simulink model "mdl_filter_kalmanIntegration_16b"  (R2016b)
settings: Solver=ode4  StartTime=0.0  StopTime=10.0  FixedStep=filterKalman_par.T  RelTol=1e-3
undefined symbols (not defined in the file or in its folder): Ag_phi_rad, Ag_theta_rad, AgVel_p_radPerScnd, AgVel_q_radPerScnd, filterKalman_par
settings Model: Creator=Nu  LastModifiedBy=Nu

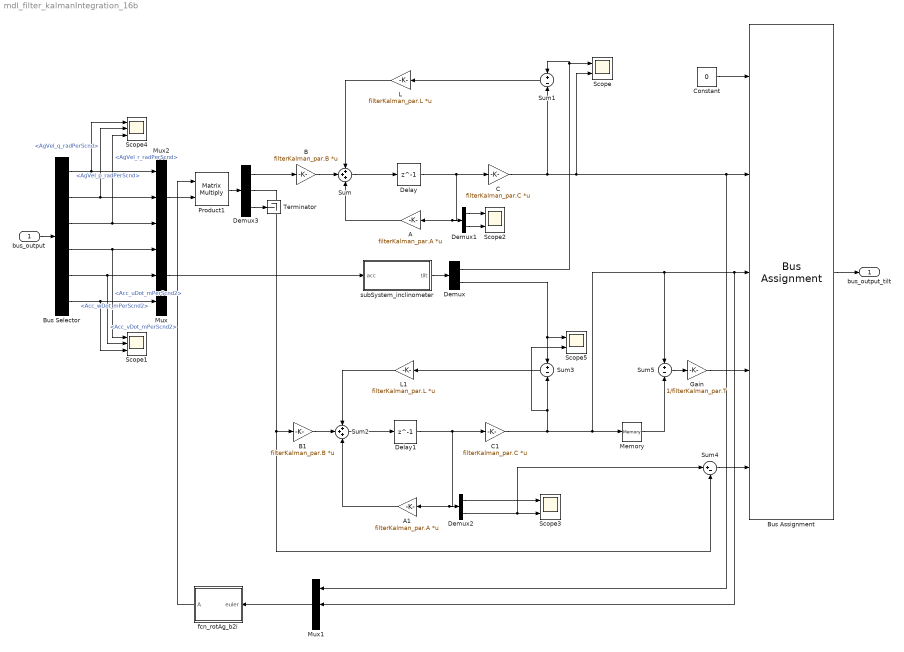
== system mdl_filter_kalmanIntegration_16b ==
  bus_output : Inport  OutDataTypeStr=Bus: mdl_output
  A : Gain  Gain=filterKalman_par.A  Multiplication=Matrix(K*u)
  A1 : Gain  Gain=filterKalman_par.A  Multiplication=Matrix(K*u)
  B : Gain  Gain=filterKalman_par.B  Multiplication=Matrix(K*u)
  B1 : Gain  Gain=filterKalman_par.B  Multiplication=Matrix(K*u)
  Bus Assignment : BusAssignment  AssignedSignals=Ag_phi_rad,Ag_theta_rad,AgVel_p_radPerScnd,AgVel_q_radPerScnd
  Bus Selector : BusSelector  OutputSignals=AgVel_p_radPerScnd,AgVel_q_radPerScnd,AgVel_r_radPerScnd,Acc_uDot_mPerScnd2,Acc_vDot_mPerScnd2,Acc_wDot_mPerScnd2
  C : Gain  Gain=filterKalman_par.C  Multiplication=Matrix(K*u)
  C1 : Gain  Gain=filterKalman_par.C  Multiplication=Matrix(K*u)
  Constant : Constant  Value=0  OutDataTypeStr=Bus: mdl_statesExt
  Delay : Delay  DelayLength=1  InitialCondition=[0 -0.014]
  Delay1 : Delay  DelayLength=1  InitialCondition=[0 -0.014]
  Demux : Demux  Outputs=2
  Demux1 : Demux  Outputs=2
  Demux2 : Demux  Outputs=2
  Demux3 : Demux  Outputs=3
  Gain : Gain  Gain=1/filterKalman_par.T
  L : Gain  Gain=filterKalman_par.L  Multiplication=Matrix(K*u)
  L1 : Gain  Gain=filterKalman_par.L  Multiplication=Matrix(K*u)
  Memory : Memory
  Mux : Mux  Inputs=3
  Mux1 : Mux  Inputs=3
  Mux2 : Mux  Inputs=3
  Product1 : Product  Multiplication=Matrix(*)
  Scope{,2..3,5} (4 alike) : Scope  NumInputPorts=2
  Scope1 : Scope  NumInputPorts=3
  Scope4 : Scope  NumInputPorts=3
  Sum : Sum  Inputs=+++
  Sum1 : Sum  Inputs=+|-
  Sum2 : Sum  Inputs=+++
  Sum3 : Sum  Inputs=+|-
  Sum4 : Sum  Inputs=|+-
  Sum5 : Sum  Inputs=+|-
  Terminator : Terminator
  fcn_rotAg_b2i : MATLAB Function  TreatAsAtomicUnit=on
  subSystem_inclinometer : Subsystem
  "bus_output_tilt " : Outport  OutDataTypeStr=Bus: mdl_statesExt
  wires:
  bus_output/1 -> Bus Selector/1
  Sum/1 -> Delay/1
  Delay/1 -> Demux1/1, A/1, C/1
  A/1 -> Sum/3
  B/1 -> Sum/2
  L/1 -> Sum/1
  Demux3/1 -> B/1
  C/1 -> Scope/2, Mux1/1, Bus Assignment/2, Sum1/2
  Sum1/1 -> L/1
  Bus Selector/4 -> Mux/1, Scope1/1  "<Acc_uDot_mPerScnd2>"
  Bus Selector/5 -> Mux/2, Scope1/2  "<Acc_vDot_mPerScnd2>"
  Bus Selector/6 -> Mux/3, Scope1/3  "<Acc_wDot_mPerScnd2>"
  Mux/1 -> subSystem_inclinometer/1(acc)
  subSystem_inclinometer/1(tilt) -> Demux/1
  Demux/1 -> Sum1/1, Scope/1
  Bus Selector/3 -> Scope4/3, Mux2/3  "<AgVel_r_radPerScnd>"
  Constant/1 -> Bus Assignment/1
  Bus Assignment/1 -> "bus_output_tilt "/1
  Demux/2 -> Scope5/1, Sum3/1
  Demux1/1 -> Scope2/1
  Demux1/2 -> Scope2/2
  Sum2/1 -> Delay1/1
  Delay1/1 -> C1/1, A1/1, Demux2/1
  A1/1 -> Sum2/3
  B1/1 -> Sum2/2
  L1/1 -> Sum2/1
  Demux3/2 -> Sum4/2, B1/1
  C1/1 -> Mux1/2, Bus Assignment/3, Sum5/1, Memory/1, Scope5/2, Sum3/2
  Sum3/1 -> L1/1
  Demux2/1 -> Scope3/1
  Demux2/2 -> Sum4/1, Scope3/2
  Sum4/1 -> Bus Assignment/5
  Sum5/1 -> Gain/1
  Memory/1 -> Sum5/2
  Gain/1 -> Bus Assignment/4
  Mux1/1 -> fcn_rotAg_b2i/1(euler)
  Mux2/1 -> Product1/2
  fcn_rotAg_b2i/1(A) -> Product1/1
  Product1/1 -> Demux3/1
  Bus Selector/1 -> Scope4/1, Mux2/1  "<AgVel_p_radPerScnd>"
  Bus Selector/2 -> Scope4/2, Mux2/2  "<AgVel_q_radPerScnd>"
  Demux3/3 -> Terminator/1

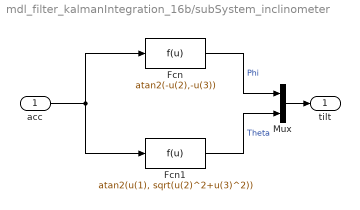
== system mdl_filter_kalmanIntegration_16b/subSystem_inclinometer ==
  acc : Inport
  Fcn : Fcn  Expr=atan2(-u(2),-u(3))
  Fcn1 : Fcn  Expr=atan2(u(1), sqrt(u(2)^2+u(3)^2))
  Mux : Mux  Inputs=2
  tilt : Outport
  wires:
  acc/1 -> Fcn/1, Fcn1/1
  Fcn/1 -> Mux/1  "Phi"
  Fcn1/1 -> Mux/2  "Theta"
  Mux/1 -> tilt/1

== matlab function mdl_filter_kalmanIntegration_16b/fcn_rotAg_b2i ==
  data: euler input; A output
function A = fcn(euler)

phi     = euler(1);
theta   = euler(2);
psi     = euler(3);

A       = mdl_rotKarman_zyx_b2i(phi, theta, psi);
